simulink model "waterTankSimulation"  (R2018a)
settings: Solver=VariableStepAuto  StartTime=0.0  StopTime=10.0  RelTol=1e-3
libraries: simulink x1
settings Model: Creator=Administrator  LastModifiedBy=Administrator

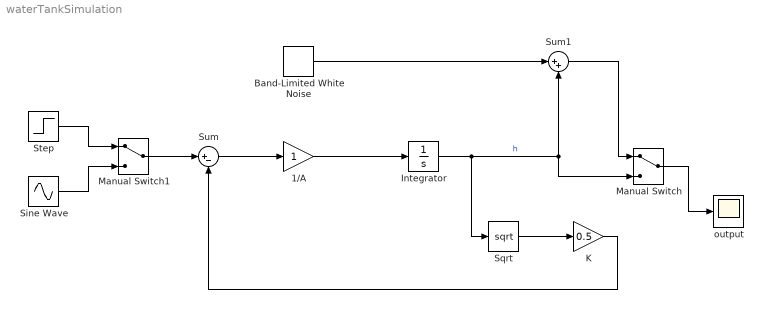
== system waterTankSimulation ==
  "1/A " : Gain
  Band-Limited White Noise : simulink/Sources/Band-Limited White Noise  Cov=[0.1]  Ts=0.1  seed=[23341]
  Integrator : Integrator
  "K " : Gain  Gain=0.5
  Manual Switch : ManualSwitch
  Manual Switch1 : ManualSwitch
  Sine Wave : Sin  SampleTime=0
  Sqrt : Sqrt  SaturateOnIntegerOverflow=on
  Step : Step  SampleTime=0
  Sum : Sum  Inputs=|+-
  Sum1 : Sum  Inputs=|++
  "output " : Scope
  wires:
  Step/1 -> Manual Switch1/1
  Sum/1 -> "1/A "/1
  "1/A "/1 -> Integrator/1
  Integrator/1 -> Sqrt/1, Manual Switch/2, Sum1/2  "h"
  Sqrt/1 -> "K "/1
  "K "/1 -> Sum/2
  Band-Limited White Noise/1 -> Sum1/1
  Sum1/1 -> Manual Switch/1
  Manual Switch/1 -> "output "/1
  Manual Switch1/1 -> Sum/1
  Sine Wave/1 -> Manual Switch1/2
